simulink model "Simulink_Lezione"  (R2020b)
settings: Solver=ode45  StartTime=0.0  StopTime=100.0  RelTol=1e-12
values from neighbouring files (symbols this model uses):
  d = 1    [symMatylab.m]
  k = 1    [symMatylab.m]
  m = 1    [symMatylab.m]
settings Model: Creator=loryb  LastModifiedBy=loryb

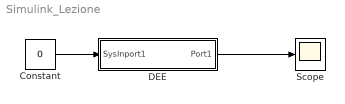
== system Simulink_Lezione ==
  Constant : Constant  Value=0
  DEE : Subsystem  mask(Differential Equation Editor (DEE)){}
      settings: OpenFcn=diffeqed
      mask Display: disp('Differential Equation\n Editor')
  Scope : Scope
  wires:
  Constant/1 -> DEE/1(SysInport1)
  DEE/1(Port1) -> Scope/1

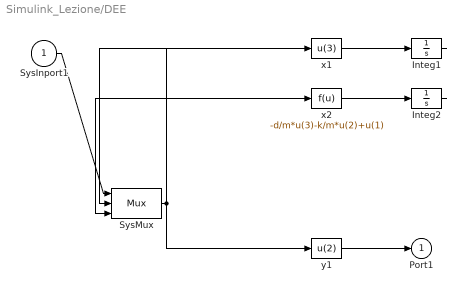
== system Simulink_Lezione/DEE ==
  SysInport1 : Inport
  Integ1 : Integrator  InitialCondition=1
  Integ2 : Integrator
  SysMux : Mux  Inputs=3
  x1 : Fcn  Expr=u(3)
  x2 : Fcn  Expr=-d/m*u(3)-k/m*u(2)+u(1)
  y1 : Fcn  Expr=u(2)
  Port1 : Outport
  wires:
  SysInport1/1 -> SysMux/1
  SysMux/1 -> x1/1, x2/1, y1/1
  x1/1 -> Integ1/1
  Integ1/1 -> SysMux/2
  x2/1 -> Integ2/1
  Integ2/1 -> SysMux/3
  y1/1 -> Port1/1
